simulink library "guidanceLawPathFollow"  (R2020a)
settings: Solver=VariableStepAuto  StartTime=0.0  StopTime=10.0  RelTol=1e-3
libraries: aileronCtrl_ul x1, calcDesTanRoll_cl x1, calcTangentialCoord_ul x1, calcTangentRollAngle_ul x1, makeOcB_cl x1, makeOcT_cl x1
settings Model: Creator=Ayaz  LastModifiedBy=Ayaz

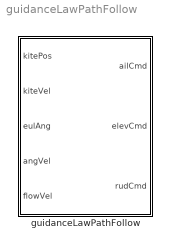
== system guidanceLawPathFollow ==
  guidanceLawPathFollow : Subsystem  mask{fltC=0}
      mask prompts: fltC "Path following controller object"

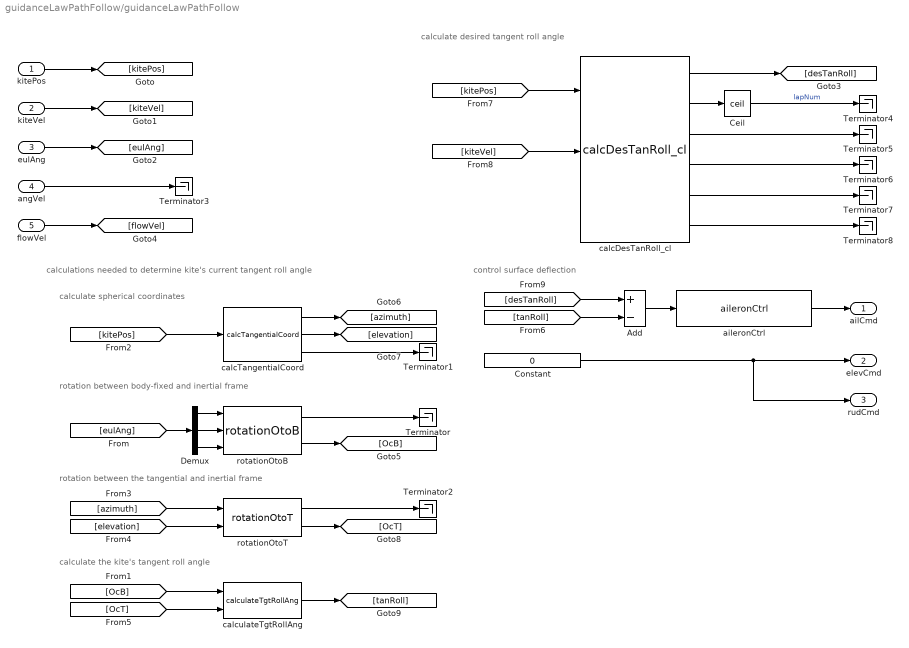
== system guidanceLawPathFollow/guidanceLawPathFollow ==
  note: calculate desired tangent roll angle
  note: control surface deflection
  note: calculations needed to determine kite's current tangent roll angle
  note: calculate the kite's tangent roll angle
  note: rotation between the tangential and inertial frame
  note: calculate spherical coordinates
  note: rotation between body-fixed and inertial frame
  kitePos : Inport
  kiteVel : Inport  Port=2
  eulAng : Inport  Port=3
  angVel : Inport  Port=4
  flowVel : Inport  Port=5
  Add : Sum  Inputs=+-
  Ceil : Rounding  Operator=ceil
  Constant : Constant  Value=0
  Demux : Demux  Outputs=3
  Terminator{,1..8} (9 alike) : Terminator
  aileronCtrl : aileronCtrl_ul/aileronCtrl  ail_kp=fltC.aileron_kp  ail_kd=fltC.aileron_kd  ail_tau=fltC.aileron_tau
  calcDesTanRoll_cl : calcDesTanRoll_cl/calcDesTanRoll_cl  fltC=fltC
  calcTangentialCoord : calcTangentialCoord_ul/calcTangentialCoord  SystemSampleTime=-1  Latency=0  AutoFrameSizeCalculation=off
  calculateTgtRollAng : calcTangentRollAngle_ul/calculateTgtRollAng  SystemSampleTime=-1  Latency=0  AutoFrameSizeCalculation=off
  rotationOtoB : makeOcB_cl/rotationOtoB  SystemSampleTime=-1  Latency=0  AutoFrameSizeCalculation=off
  rotationOtoT : makeOcT_cl/rotationOtoT  SystemSampleTime=-1  Latency=0  AutoFrameSizeCalculation=off
  ailCmd : Outport
  elevCmd : Outport  Port=2
  rudCmd : Outport  Port=3
  wires:
  kitePos/1 -> [kitePos]
  kiteVel/1 -> [kiteVel]
  eulAng/1 -> [eulAng]
  angVel/1 -> Terminator3/1
  flowVel/1 -> [flowVel]
  Demux/2 -> rotationOtoB/2
  Demux/1 -> rotationOtoB/1
  Demux/3 -> rotationOtoB/3
  [eulAng] -> Demux/1
  rotationOtoB/2 -> [OcB]
  [OcB] -> calculateTgtRollAng/1
  rotationOtoB/1 -> Terminator/1
  [kitePos] -> calcTangentialCoord/1
  calcTangentialCoord/1 -> [azimuth]
  calcTangentialCoord/2 -> [elevation]
  calcTangentialCoord/3 -> Terminator1/1
  [azimuth] -> rotationOtoT/1
  [elevation] -> rotationOtoT/2
  rotationOtoT/2 -> [OcT]
  rotationOtoT/1 -> Terminator2/1
  [OcT] -> calculateTgtRollAng/2
  calculateTgtRollAng/1 -> [tanRoll]
  [kitePos] -> calcDesTanRoll_cl/1
  [kiteVel] -> calcDesTanRoll_cl/2
  calcDesTanRoll_cl/1 -> [desTanRoll]
  [desTanRoll] -> Add/1
  [tanRoll] -> Add/2
  Add/1 -> aileronCtrl/1
  aileronCtrl/1 -> ailCmd/1
  Constant/1 -> rudCmd/1, elevCmd/1
  calcDesTanRoll_cl/2 -> Ceil/1
  calcDesTanRoll_cl/3 -> Terminator5/1
  calcDesTanRoll_cl/5 -> Terminator7/1
  calcDesTanRoll_cl/4 -> Terminator6/1
  calcDesTanRoll_cl/6 -> Terminator8/1
  Ceil/1 -> Terminator4/1  "lapNum"
